simulink model "airframeOpenLoop"  (R2019a)
settings: Solver=VariableStepAuto  StartTime=0.0  StopTime=50  RelTol=1e-3
settings Model: Creator=tdarrah  LastModifiedBy=darrahts
settings DataIOCC: ReturnWorkspaceOutputs=off
settings DebuggingCC: ArithmeticOperatorsInVariantConditions=warning
settings SFSimCC: SimUseLocalCustomCode=off
settings RTWCC: RTWUseLocalCustomCode=off
settings CodeAppCC: StateflowObjectComments=on

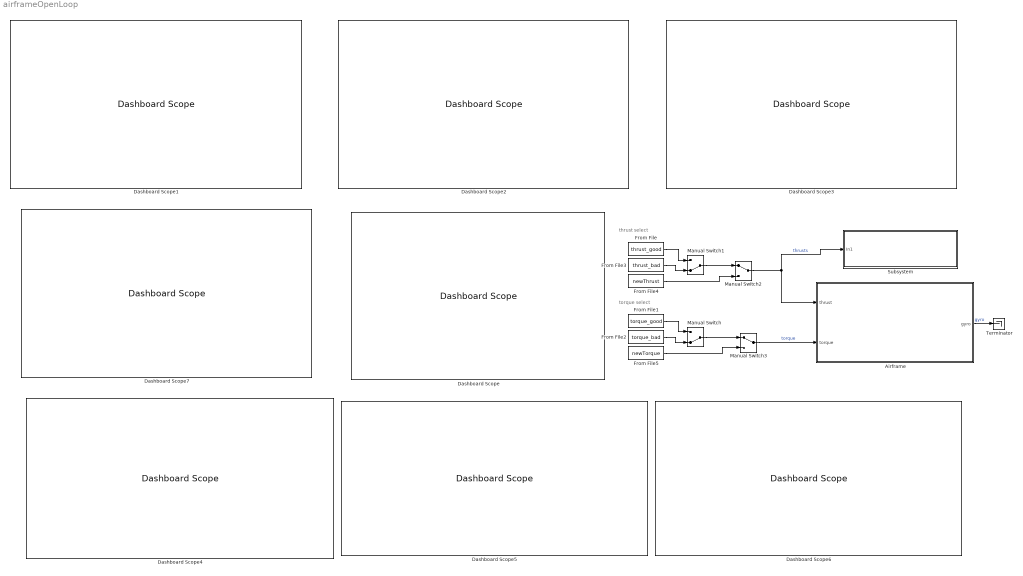
== system airframeOpenLoop ==
  note: thrust select
  note: torque select
  Airframe : Subsystem
  Dashboard Scope{,1..7} (8 alike) : DashboardScope
  From File : FromFile  FileName=thrust_good
  From File1 : FromFile  FileName=torque_good
  From File2 : FromFile  FileName=torque_bad
  From File3 : FromFile  FileName=thrust_bad
  From File4 : FromFile  FileName=newThrust
  From File5 : FromFile  FileName=newTorque
  Manual Switch : ManualSwitch  CurrentSetting=0
  Manual Switch1 : ManualSwitch  CurrentSetting=0
  Manual Switch2 : ManualSwitch
  Manual Switch3 : ManualSwitch
  Subsystem : Subsystem
  Terminator : Terminator
  wires:
  Manual Switch1/1 -> Manual Switch2/1
  From File/1 -> Manual Switch1/1
  From File1/1 -> Manual Switch/1
  Manual Switch/1 -> Manual Switch3/1
  From File2/1 -> Manual Switch/2
  From File3/1 -> Manual Switch1/2
  Airframe/1(gyro) -> Terminator/1  "gyro"
  Manual Switch2/1 -> Subsystem/1(In1), Airframe/1(thrust)  "thrusts"
  Manual Switch3/1 -> Airframe/2(torque)  "torque"
  From File4/1 -> Manual Switch2/2
  From File5/1 -> Manual Switch3/2

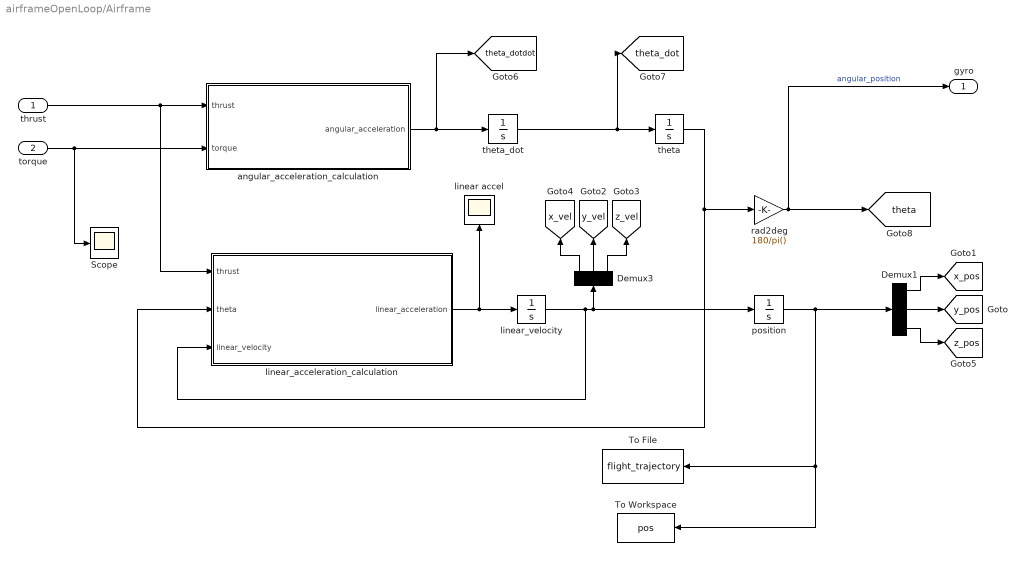
== system airframeOpenLoop/Airframe ==
  thrust : Inport
  torque : Inport  Port=2
  Demux1 : Demux  Outputs=3
  Demux3 : Demux  Outputs=3
  Scope : Scope
  To File : ToFile  Filename=flight_trajectory  MatrixName=pos  SampleTime=.1
  To Workspace : ToWorkspace  VariableName=pos  SampleTime=-1
      settings: Save2DSignal=2-D array (concatenate along first dimension)
  angular_acceleration_calculation : MATLAB Function  TreatAsAtomicUnit=on
  linear accel : Scope
  linear_acceleration_calculation : MATLAB Function  TreatAsAtomicUnit=on
  linear_velocity : Integrator
  "position " : Integrator
  rad2deg : Gain  Gain=180/pi()
  theta : Integrator
  theta_dot : Integrator
  gyro : Outport
  tag scope: theta=global, theta_dot=global, theta_dotdot=global, x_pos=global, x_vel=global, y_pos=global, y_vel=global, z_pos=global, z_vel=global
  wires:
  Demux1/1 -> [x_pos]
  rad2deg/1 -> [theta], gyro/1  "angular_position"
  Demux1/3 -> [z_pos]
  Demux1/2 -> [y_pos]
  linear_acceleration_calculation/1(linear_acceleration) -> linear_velocity/1, linear accel/1
  Demux3/2 -> [y_vel]
  torque/1 -> Scope/1, angular_acceleration_calculation/2(torque)
  thrust/1 -> linear_acceleration_calculation/1(thrust), angular_acceleration_calculation/1(thrust)
  theta_dot/1 -> [theta_dot], theta/1
  Demux3/3 -> [z_vel]
  "position "/1 -> Demux1/1, To File/1, To Workspace/1
  angular_acceleration_calculation/1(angular_acceleration) -> [theta_dotdot], theta_dot/1
  theta/1 -> rad2deg/1, linear_acceleration_calculation/2(theta)
  Demux3/1 -> [x_vel]
  linear_velocity/1 -> Demux3/1, "position "/1, linear_acceleration_calculation/3(linear_velocity)

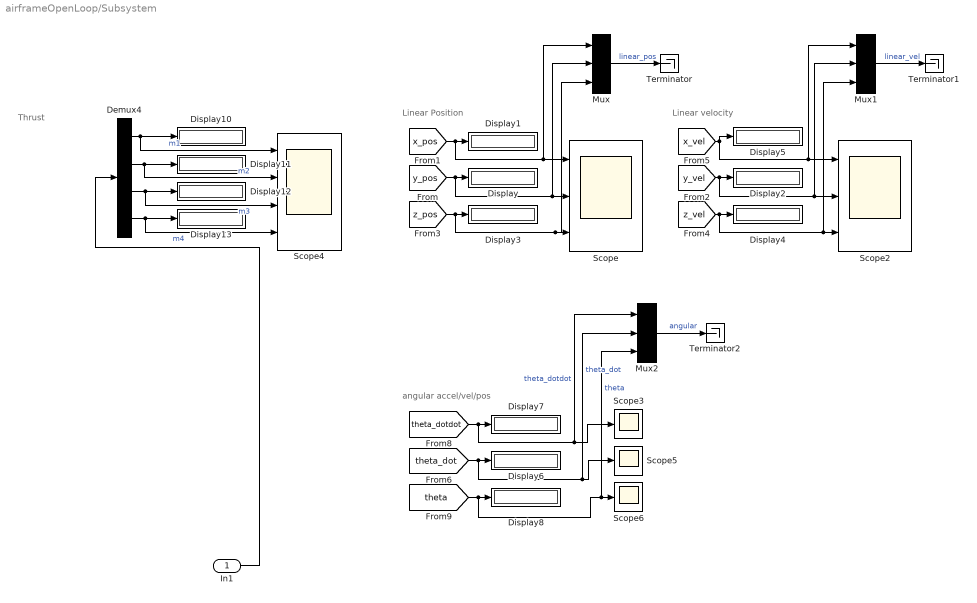
== system airframeOpenLoop/Subsystem ==
  note: Linear velocity
  note: Linear Position
  note: Thrust
  note: angular accel/vel/pos
  In1 : Inport
  Demux4 : Demux
  Display{,1..8,10..13} (13 alike) : Display
  Mux : Mux  Inputs=3
  Mux1 : Mux  Inputs=3
  Mux2 : Mux  Inputs=3
  Scope : Scope  NumInputPorts=3
  Scope2 : Scope  NumInputPorts=3
  Scope3 : Scope
  Scope4 : Scope  NumInputPorts=4
  Scope5 : Scope
  Scope6 : Scope
  Terminator : Terminator
  Terminator1 : Terminator
  Terminator2 : Terminator
  wires:
  [y_pos] -> Mux/2, Scope/2, Display/1
  Demux4/4 -> Scope4/4, Display13/1  "m4"
  [z_pos] -> Mux/3, Scope/3, Display3/1
  [x_pos] -> Mux/1, Scope/1, Display1/1
  Demux4/1 -> Scope4/1, Display10/1  "m1"
  In1/1 -> Demux4/1
  Demux4/2 -> Scope4/2, Display11/1  "m2"
  Demux4/3 -> Scope4/3, Display12/1  "m3"
  Mux/1 -> Terminator/1  "linear_pos"
  [y_vel] -> Mux1/2, Scope2/2, Display2/1
  [z_vel] -> Mux1/3, Scope2/3, Display4/1
  [x_vel] -> Mux1/1, Scope2/1, Display5/1
  Mux1/1 -> Terminator1/1  "linear_vel"
  [theta_dot] -> Mux2/2, Scope5/1, Display6/1  "theta_dot"
  [theta] -> Mux2/3, Scope6/1, Display8/1  "theta"
  [theta_dotdot] -> Mux2/1, Scope3/1, Display7/1  "theta_dotdot"
  Mux2/1 -> Terminator2/1  "angular"

== matlab function airframeOpenLoop/Airframe/angular_acceleration_calculation ==
  data: thrust input; torque input; angular_acceleration output
function angular_acceleration = calc_angular_acceleration(thrust, torque)
%
% inputs: torque vector
%         thrust vector
%
% output: rotational acceleration (of drone)
%

% moments about each axis (x,y,z) i.e. (pitch, roll, yaw)
moments = [0 0 0];

% rotational acceleration about each axis
angular_acceleration = [0 0 0];

% moments of inertia empirically derived from sample data
moments_I = [.003, .003, .007];

% pitch
% motor pair A * 1/2 rigid body length - motor pair B * rigid body length
moments(1) = (thrust(3) + thrust(4))*.237/2 - (thrust(1)+thrust(2))*.237/2;
% roll
% motor pair A * 1/2 rigid body length - motor pair B * rigid body length
moments(2) = (thrust(3) + thrust(2))*.237/2 - (thrust(1)+thrust(4))*.237/2;
%yaw
% motor pair A - motor pair B
moments(3) = (torque(4) + torque(2)) - (torque(1)  + torque(3));

for i=1:3
    angular_acceleration(i) = moments(i) / moments_I(i);
end

== matlab function airframeOpenLoop/Airframe/linear_acceleration_calculation ==
  data: thrust input; linear_acceleration output; theta input; linear_velocity input
function linear_acceleration = calc_linear_acceleration(thrust,theta, linear_velocity)
%
% inputs: thrust vector (m1, m2, m3, m4)
%         disturbances vector (x,y,z)
%         theta vector (x,y,z)
%         linear velocity vector (x,y,z)
%
% output: linear acceleration vector (x,y,z)
%
disturbances = [0.0 0.0 0.0 0.0];

m = .743; % mass of drone
g = 9.81; % acceleration due to gravity
rho = 1.225; % density of air at sea level
coef_d = 1.0; % coefficient of drag for the drone

% cross sectional areas of drone in x,y,z planes
areas = [.0197, .0197, .0512];

linear_acceleration = [0 0 0];
force = [0 0 0];
xyz_thrust = [0;0;0];
drag = [0 0 0];

% trigonometric functions for calculating pitch,roll,yaw (x,y,z) thrust 
xyz_thrust(1,1) = sin(theta(2))*cos(theta(1))*sum(thrust);
xyz_thrust(2,1) = sin(theta(1))*cos(theta(2))*sum(thrust);
xyz_thrust(3,1) = cos(theta(1))*cos(theta(2))*sum(thrust);

% angular position and magnitude on the pitch-roll (x,y) plane
angular_pos =-atan2(xyz_thrust(1), xyz_thrust(2));
angular_mag = sqrt(xyz_thrust(1)^2 + xyz_thrust(2)^2);

% if the drone is pointed upwards, x and y thrust uses + theta(3) (z)
if(xyz_thrust(3) >= 0)
    xyz_thrust(1) = angular_mag * sin(angular_pos + theta(3));
    xyz_thrust(2) = angular_mag * cos(angular_pos + theta(3));
else
    xyz_thrust(1) = angular_mag * sin(angular_pos - theta(3));
    xyz_thrust(2) = angular_mag * cos(angular_pos - theta(3));  
end

% calculate drage and force in x,y,z 
for i=1:3
    drag(i) = .5*rho*linear_velocity(i)^2* areas(i)*coef_d;
    % if the drone is going backward (w.r.t its local coordinate system)
    if (linear_velocity(i) < 0)
        force(i) = xyz_thrust(i) - disturbances(i) + drag(i);
    else
        force(i) = xyz_thrust(i) - disturbances(i) - drag(i);
    end
    % account for gravity in the z direction
    if(i == 3)
        force(i) = force(i) - m*g;
    end
end

%f=ma to calculate final acceleration
for i=1:3
    linear_acceleration(i) = force(i)/m;
end
